simulink model "doc_ortho"  (R2014a)
settings: Solver=FixedStepDiscrete  StartTime=0.0  StopTime=127  RelTol=1e-3
libraries: commseqgen2 x3, simulink x1
settings Model: Creator=The MathWorks Inc.
settings DataIOCC: SignalLoggingSaveFormat=ModelDataLogs  SignalLoggingName=sigsOut
settings OptimizationCC: BooleanDataType=off  ExpressionDepthLimit=2147483647
settings DebuggingCC: SaveWithParameterizedLinksMsg=none  UnderspecifiedInitializationDetection=Classic  SolverPrmCheckMsg=none  MultiTaskDSMMsg=warning  MultiTaskCondExecSysMsg=none  FcnCallInpInsideContextMsg=UseLocalSettings  StateNameClashWarn=warning  StrictBusMsg=None
settings HardwareCC: ProdHWDeviceType=Specified
settings RTWCC: IncludeERTFirstTime=on
settings CodeAppCC: MangleLength=5
settings GRTTargetCC: TargetFcnLib=iso_c_tmw.mat  CombineOutputUpdateFcns=off  GRTInterface=on

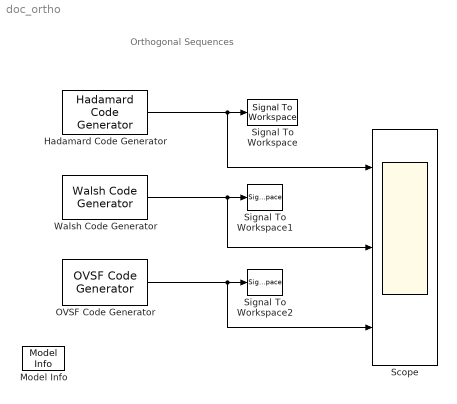
== system doc_ortho ==
  note: Orthogonal Sequences
  Hadamard Code Generator : commseqgen2/Hadamard Code Generator  length=64  index=31  ts=1  frameBased=off  sampPerFrame=1  outDataType=double
  Model Info : simulink/Model-Wide Utilities/Model Info  InitialBlockCM=None  BlockCM=None  Frame=on  DisplayStringWithTags=Info  HorizontalTextAlignment=Center  LeftAlignmentValue=0.5  SourceBlockDiagram=doc_ortho  TagMaxNumber=20
  OVSF Code Generator : commseqgen2/OVSF Code Generator  spreadFact=64  index=31  ts=1  frameBased=off  sampPerFrame=1  outDataType=double
  Scope : Scope  NumInputPorts=3
      settings: YMin=-1.5~-1.5~-1.5  YMax=1.5~1.5~1.5
  Signal To Workspace : SignalToWorkspace  VariableName=had
      settings: CopyFcn=dspblkcopystw(gcbh);  Save2DSignal=3-D array (concatenate along third dimension)
  Signal To Workspace1 : SignalToWorkspace  VariableName=walsh
      settings: CopyFcn=dspblkcopystw(gcbh);  Save2DSignal=3-D array (concatenate along third dimension)
  Signal To Workspace2 : SignalToWorkspace  VariableName=ovsf
      settings: CopyFcn=dspblkcopystw(gcbh);  Save2DSignal=3-D array (concatenate along third dimension)
  Walsh Code Generator : commseqgen2/Walsh Code Generator  length=64  index=31  ts=1  frameBased=off  sampPerFrame=1  outDataType=double
  wires:
  Hadamard Code Generator/1 -> Signal To Workspace/1, Scope/1
  Walsh Code Generator/1 -> Signal To Workspace1/1, Scope/2
  OVSF Code Generator/1 -> Signal To Workspace2/1, Scope/3
